simulink library "gbt_library"  (Simulink 7.4)
settings: Solver=ode45  StartTime=0.0  StopTime=10.0  RelTol=1e-3
libraries: xbsIndex_r4 x1525, casper_library_flow_control x20, casper_library_misc x15, xps_library x1
(part 1 of 14)
settings Model: Creator=mwagner  LastModifiedBy=chenhong

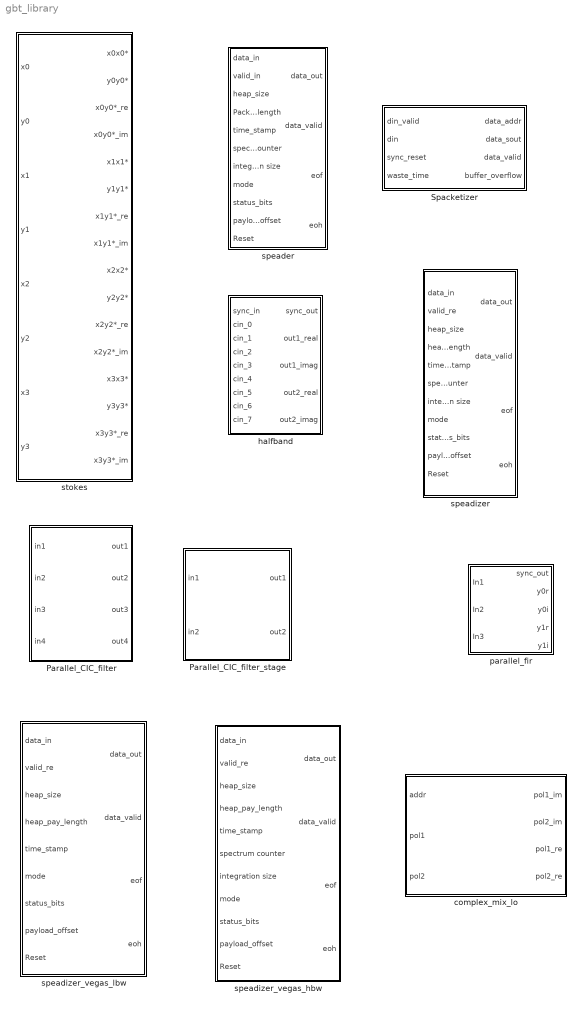
== system gbt_library ==
  Parallel_CIC_filter : Subsystem  mask(Parallel_CIC_filter){n_stages=3, dec_rate=6, n_inputs=4, polyphase=off, add_latency=1, n_bits=8, bin_pt=7, dec2_halfout=off, half2first=off, recursives=[0 1 1 1], reduced_crtc_path=off}
      mask prompts: n_stages "CIC filter Order"; dec_rate "Decimation rate"; n_inputs "Number of inputs"; polyphase "polyphase structure?(Effective only when n_inputs = 1 or n_inputs = dec_rate)"; add_latency "Add latency"; n_bits "Input bit width"; bin_pt "Binary point"; dec2_halfout "When dec_rate =2, half the number of outputs?"; half2first "Order of stages: Smaller prime factors first?"; recursives "Recursive structure for each prime-factor stage"; reduced_crtc_path "In recursive stages, invoke reduced critical path structure?"
      mask help:
      | A non-recursive CIC filter with parallel inputs.
      | Decimation rate is factored into prime numbers. Each implemented using a single stage.
      |
      | Expecting a 1-dimensional boolean vector for
      | choosing the recursive/nonrecursive structure of each prime-factor stage.
      | ([0 1 1 0] means [non-recursive recursive recursive non-recursive] stages.)
      |
      | For each stages:
      | Only supports decimation rate that is a prime number.
      | If dec_rate = 2, then we can choose n_outputs = 0.5*n_inputs(less resource)
      |     or n_outputs = n_inputs.
      | In other cases, n_outputs = n_inputs.
      | Polyphase structure available for stages of n_inputs is 1 or 2.
      mask init:
      | config.source = str2func('parallel_cic_filter_init_xblock');
      | config.toplevel = gcb;
      | config.depend = get_dependlist('parallel_cic_filter'); 
      | set_param(gcb,'LinkStatus','inactive');
      | xBlock(config, {config.toplevel,...
      |                 'n_stages',n_stages, ...
      |                 'dec_rate', dec_rate, ...
      |                 'n_inputs', n_inputs,...
      |                 'polyphase', polyphase,...
      |                 'add_latency',add_latency,...
      |                 'dec2_halfout', dec2_halfout, ...
      |                 'half2first', half2first,...
      |                 'n_bits', n_bits, ...
      |                 'bin_pt', bin_pt,...
      |                 'reduced_crtc_path', reduced_crtc_path, ...
      |                 'recursives', recursives} ...
      |                 );
      | disp('new block added');
      settings: AttributesFormatString=|
      | dec_rate = 6
      | Order = 3
  Parallel_CIC_filter_stage : Subsystem  mask(Parallel_CIC_filter_stage){n_stages=3, dec_rate=3, n_inputs=2, polyphase=off, add_latency=1, n_bits=8, bin_pt=7, dec2_halfout=on, recursive=on, reduced_crtc_path=on}
      mask prompts: n_stages "CIC filter Order"; dec_rate "Decimation rate"; n_inputs "Number of Inputs"; polyphase "polyphase structure?(Effective only when n_inputs = 1 or n_inputs = dec_rate)"; add_latency "Add latency"; n_bits "Input bit width"; bin_pt "Binary point"; dec2_halfout "When dec_rate =2, half the number of outputs?"; recursive "Recursive Structure?"; reduced_crtc_path "In recursive stages, invoke reduced critical path structure?"
      mask help:
      | A single stage of CIC filter with parallel inputs.
      | Only supports decimation rate that is a prime number.
      | If dec_rate = 2, then n_outputs = 0.5*n_inputs.
      | In other cases, n_outputs = n_inputs.
      | Polyphase structure available when n_inputs is 1 or 2.
      mask init:
      | config.source=str2func('parallel_polynomial_dec_stage_init_xblock');
      | config.toplevel=gcb;
      | config.depend = get_dependlist('parallel_polynomial_dec_stage');
      | set_param(gcb,'LinkStatus','inactive');
      | xBlock(config, {config.toplevel, ...
      |                 'n_stages', n_stages, ...
      |                 'dec_rate', dec_rate, ...
      |                 'n_inputs', n_inputs, ...
      |                 'polyphase', polyphase, ...
      |                 'add_latency', add_latency, ...
      |                 'n_bits', n_bits, ...
      |                 'bin_pt', bin_pt, ...
      |                 'dec2_halfout', dec2_halfout, ...
      |                 'recursive', recursive, ...
      |                 'reduced_crtc_path', reduced_crtc_path});
      settings: AttributesFormatString=|
      | recursive
      |  8_in
      |  reducded critical path: off
      mask CallbackString:
      | |n=get_param(gcb,'dec_rate');
      | if ~isempty(n)
      |     n = eval(n);
      |     if ~isprime(n)
      |         errordlg('Only supports decimation rate that is a prime number');
      |         set_param(gcb,'dec_rate','');
      |     end
      | end||||||||
  Spacketizer : Subsystem  AncestorBlock=gbt_library/packetizer  mask(packetizer){pin_width=256, sout_width=64, fifo_depth=128, total_words=32}
      mask prompts: pin_width "Parallel Input Width"; sout_width "Serial Output Width"; fifo_depth "FIFO depth"; total_words "Total number of data points"
      mask help:
      | This block is intended to serialize data that is 'bursty', that is,
      | the average data rate is small but per cycle the data is highly
      | parallel and can contain many points simultaneously.  This situation
      | is common with the streaming CASPER FFTs and related blocks.
      |
      | The serialization buffers the data when valid and independently
      | serializes the data when the buffer is non-empty.  For convenience, the
      | data is counted as it is serialized and signals exist to indicate
      | that the serial output is valid or that a buffer overflow has occured.  The
      | block will not stop in the case of an overflow, and the overflow
      | signal is not held high after it occurs.
      |
      | For example usage, see 'roach_spec_2adc_borph' in 'SVNROOT/trunk/projects/roach_spec/'
      | or the test case in 'SVNROOT/trunk/mlib_devel_10_1/Tests/packetizer_test.mdl'
      |
      | For extended documentation, please see the CASPER wiki
      mask init:
      | packetizer_init(gcb, 'pin_width', pin_width, 'sout_width', sout_width, 'total_words', total_words, 'fifo_depth', fifo_depth)
      | % packetizer_init(gcb, ...
      | %     'pin_width', pin_width, ...
      | %     'sout_width', sout_width, ...
      | %   %  'fifo_depth', fifo_depth, ...
      | %     'total_words', total_words);
      settings: AttributesFormatString=|
      | Parallel Input Width: 256
      | Serial Output Width: 64
      mask StyleString: edit,edit,popup(16|32|64|128|256|512|1K|2K|4K|8K|16K|32K|64K),edit
  complex_mix_lo : Subsystem  AncestorBlock=gbt_library/complex_mix_lo
  halfband : Subsystem  mask(halfband filter){ExplicitCoefficient=off, filter_coeffs=0, n_taps=4, window=hamming}
      mask prompts: ExplicitCoefficient "Explicitly define coefficients?"; filter_coeffs "Filter Coefficients"; n_taps "Number of Taps (FIR order)"; window "Window Type"
      mask help: A halfband filter for 8 complex inputs
      mask init:
      | config.source = str2func('half_band_init_xblock');
      | config.depend = get_dependlist('half_band');
      | config.debug = 0;
      | config.toplevel = gcb;
      | disp('hey');
      | ExplicitCoefficient
      | filter_coeffs
      | n_taps
      | window
      | xBlock(config, {config.toplevel, ...
      |                  'ExplicitCoefficient', ExplicitCoefficient, ...
      |                  'filter_coeffs', filter_coeffs, ...
      |                  'n_taps', n_taps, ...
      |                  'window', window, ...
      |     });
      mask Help: eval('xlWeb(''http://casper.berkeley.edu/wiki/halfband'')')
      mask StyleString: checkbox,edit,edit,popup(hamming|chebwin|gausswin|kaiserwin)
      mask CallbackString:
      | e_c = get_param(gcb, 'ExplicitCoefficient');
      | if strcmp(e_c, 'off')
      |     n_e_c = 'on';
      | else
      |     n_e_c = 'off';
      | end
      | set_param_state(gcb, 'filter_coeffs', e_c);
      | set_param_state(gcb, 'n_taps', n_e_c);
      | set_param_state(gcb, 'window', n_e_c);|||
  parallel_fir : Subsystem  mask(Parallel FIR Filter){filter_coeffs=[1 2 3 4 5 6 7 8]}
      mask prompts: filter_coeffs "Filter coefficients"
      mask help: Xblock
      mask init:
      | config.source=str2func('parallel_fir_init_xblock');
      | config.toplevel=gcb;
      | config.depend = get_dependlist('parallel_fir');
      | set_param(gcb,'LinkStatus','inactive');
      | xBlock(config, ...
      |         {config.toplevel, filter_coeffs})
      mask CallbackString:
      | filter_coeffs = get_param(gcb,'filter_coeffs');
      | if ~isempty(filter_coeffs)
      |     filter_coeffs = eval(filter_coeffs);
      |     if parallel_fir_coefficient_check(filter_coeffs)
      |         set_param(gcb,'filter_coeffs','');
      |     end
      | end
  speader : Subsystem  AncestorBlock=gbt_library/spead_packet  mask{spead_msw=64, spead_lsw=40, num_items=6, num_payloads=2}
      mask prompts: num_items "Number of items (+5)"; num_payloads "number of payloads"
      mask help:
      | The size of the heap and payload are in Bytes.
      | If there is one packet per heap then payload_offset is 0.
      | All the input must be not longer than 40 bits.
  speadizer : Subsystem  AncestorBlock=gbt_library/spead_packet  mask{spead_msw=64, spead_lsw=40, num_items=6, num_payloads=2}
      mask prompts: num_items "Number of items (+5)"; num_payloads "number of payloads"
      mask help:
      | The size of the heap and payload are in Bytes.
      | If there is one packet per heap then payload_offset is 0.
      | All the input must be not longer than 40 bits.
  speadizer_vegas_hbw : Subsystem  AncestorBlock=gbt_library/speadizer  mask(speadizer_vegas){spead_msw=64, spead_lsw=40, num_items=6, num_payloads=2, pktzr_waste_time=7, data_input_width=512}
      mask prompts: spead_msw "Num bits for SPEAD Item ID"; spead_lsw "Num bits for SPEAD Item value"; num_items "Number of items (+5)"; num_payloads "Number of packets per heap"; pktzr_waste_time "Packetizer waste time"; data_input_width "Data input width"
      mask help:
      | The size of the heap and payload are in Bytes.
      | If there is one packet per heap then payload_offset is 0.
      | All the input must be not longer than 40 bits.
      mask init:
      | speadizer_vegas_init(gcb, 'spead_msw', spead_msw, 'spead_lsw', spead_lsw, 'num_items', num_items, 'num_payloads', num_payloads, 'pktzr_waste_time', pktzr_waste_time, 'data_input_width', data_input_width)
  speadizer_vegas_lbw : Subsystem  mask(speadizer_vegas){spead_msw=24, spead_lsw=40, num_items=4, num_payloads=1, pktzr_waste_time=0, data_input_width=256}
      mask prompts: spead_msw "Num bits for SPEAD Item ID"; spead_lsw "Num bits for SPEAD Item value"; num_items "Number of items (+5)"; num_payloads "Number of packets per heap"; pktzr_waste_time "Packetizer waste time"; data_input_width "Data input width"
      mask help:
      | The size of the heap and payload are in Bytes.
      | If there is one packet per heap then payload_offset is 0.
      | All the input must be not longer than 40 bits.
      mask init: same as gbt_library/speadizer_vegas_hbw
  stokes : Subsystem  mask{n_samples=4}
      mask prompts: n_samples "Number of Simultaneous Inputs"
      mask init:
      | % To make the xBlock smart so it won''t re-generate the
      | % subsystem if neither the arguments nor the scripts are
      | % changes, use as the following:
      | cfg.source = str2func('stokes_init');
      | cfg.toplevel = gcb;
      | cfg.depend = {'stokes_init'};
      | args = {n_samples};
      | xBlock(cfg, args);
      mask TabNameString: Basic

== system gbt_library/Parallel_CIC_filter ==
  in1 : Inport
  in2 : Inport  Port=2
  in3 : Inport  Port=3
  in4 : Inport  Port=4
  Stage1_dec3 : Subsystem
      settings: AttributesFormatString=|
      | nonrecursive
      | 8_in
      | polyphase:off
  Stage2_dec2 : Subsystem
      settings: AttributesFormatString=|
      | recursive
      | 13_in
      | reduced critical path structureoff
  out1 : Outport
  out2 : Outport  Port=2
  out3 : Outport  Port=3
  out4 : Outport  Port=4
  wires:
  Stage2_dec2/4(out4) -> out4/1
  Stage2_dec2/3(out3) -> out3/1
  Stage2_dec2/2(out2) -> out2/1
  Stage2_dec2/1(out1) -> out1/1
  Stage1_dec3/4(out4) -> Stage2_dec2/4(in4)  "sig2_4"
  Stage1_dec3/3(out3) -> Stage2_dec2/3(in3)  "sig2_3"
  Stage1_dec3/2(out2) -> Stage2_dec2/2(in2)  "sig2_2"
  Stage1_dec3/1(out1) -> Stage2_dec2/1(in1)  "sig2_1"
  in4/1 -> Stage1_dec3/4(in4)
  in3/1 -> Stage1_dec3/3(in3)
  in2/1 -> Stage1_dec3/2(in2)
  in1/1 -> Stage1_dec3/1(in1)

== system gbt_library/Parallel_CIC_filter_stage ==
  in1 : Inport
  in2 : Inport  Port=2
  comb_1 : Subsystem
      settings: AttributesFormatString=|
      | Differentiation length = 1
      | Bitwidth = 13 bin_pt=7
  comb_2 : Subsystem
      settings: AttributesFormatString=|
      | Differentiation length = 1
      | Bitwidth = 13 bin_pt=7
  comb_3 : Subsystem
      settings: AttributesFormatString=|
      | Differentiation length = 1
      | Bitwidth = 13 bin_pt=7
  downsample_3 : Subsystem
      settings: AttributesFormatString=Decimation Rate = 3
  int_1 : Subsystem
      settings: AttributesFormatString=|
      | Add Latency = 1
      | Bitwidth = 13 bin_pt = 7
  int_2 : Subsystem
      settings: AttributesFormatString=|
      | Add Latency = 1
      | Bitwidth = 13 bin_pt = 7
  int_3 : Subsystem
      settings: AttributesFormatString=|
      | Add Latency = 1
      | Bitwidth = 13 bin_pt = 7
  out1 : Outport
  out2 : Outport  Port=2
  wires:
  in1/1 -> downsample_3/1(sync_in), int_1/3(sync), int_1/1(in1)
  int_1/1(out1) -> int_2/3(sync), int_2/1(in1)  "int_ins1_1"
  int_2/1(out1) -> int_3/3(sync), int_3/1(in1)  "int_ins2_1"
  comb_3/3(out2) -> out2/1  "comb_ins3_2"
  comb_3/2(out1) -> out1/1  "comb_ins3_1"
  comb_2/3(out2) -> comb_3/3(in2)  "comb_ins2_2"
  comb_2/2(out1) -> comb_3/2(in1)  "comb_ins2_1"
  comb_2/1(sync_out) -> comb_3/1(sync_in)  "comb_sync_in3"
  comb_1/3(out2) -> comb_2/3(in2)  "comb_ins1_2"
  comb_1/2(out1) -> comb_2/2(in1)  "comb_ins1_1"
  comb_1/1(sync_out) -> comb_2/1(sync_in)  "comb_sync_in2"
  downsample_3/3(Out2) -> comb_1/3(in2)  "ds_out2"
  downsample_3/2(Out1) -> comb_1/2(in1)  "ds_out1"
  downsample_3/1(sync_out) -> comb_1/1(sync_in)  "ds_sync_out"
  int_3/2(out2) -> downsample_3/3(In2)  "int_ins3_2"
  int_3/1(out1) -> downsample_3/2(In1)  "int_ins3_1"
  int_2/2(out2) -> int_3/2(in2)  "int_ins2_2"
  int_1/2(out2) -> int_2/2(in2)  "int_ins1_2"
  in2/1 -> int_1/2(in2)

== system gbt_library/Spacketizer ==
  din_valid : Inport
  din : Inport  Port=2
  sync_reset : Inport  Port=3
  waste_time : Inport  Port=4
  Counter : xbsIndex_r4/Counter  cnt_type=Free Running  cnt_to=Inf  operation=Up  start_count=0  cnt_by_val=1  arith_type=Unsigned  n_bits=11  bin_pt=0  load_pin=off  rst=on  en=on  explicit_period=on  period=1  dbl_ovrd=off  use_behavioral_HDL=off  implementation=Fabric  use_rpm=off  block_type=counter
  Inverter : xbsIndex_r4/Inverter  en=off  latency=0  dbl_ovrd=off  block_type=inv
  Logical : xbsIndex_r4/Logical  logical_function=AND  inputs=2  en=off  latency=0  precision=Full  arith_type=Unsigned  n_bits=16  bin_pt=0  align_bp=on  dbl_ovrd=off  block_type=logical
  Logical1 : xbsIndex_r4/Logical  logical_function=AND  inputs=2  en=off  latency=0  precision=Full  arith_type=Unsigned  n_bits=16  bin_pt=0  align_bp=on  dbl_ovrd=off  block_type=logical
  data_buffer : xbsIndex_r4/FIFO  depth=128  percent_nbits=1  rst=off  en=off  use_dcount=off  use_almost_empty=off  almost_empty_thresh=2  use_almost_full=off  almost_full_thresh=14  dbl_ovrd=off  mem_type=Block RAM  explicit_period=off  block_type=fifo
      settings: block_version=10.1.3
  data_counter : xbsIndex_r4/Counter  cnt_type=Free Running  cnt_to=Inf  operation=Up  start_count=0  cnt_by_val=1  arith_type=Unsigned  n_bits=6  bin_pt=0  load_pin=off  rst=on  en=on  explicit_period=on  period=1  dbl_ovrd=off  use_behavioral_HDL=off  implementation=Fabric  use_rpm=off  block_type=counter
  packetizer_fsm : xbsIndex_r4/MCode  mfname=packetizer_fsm  explicit_period=off  period=1  inputsTable={'boundInpExpr'=>['','','3','','31','','',''],'inputs'=>['fifo_empty','shift_count','data_per_word','data_count','n_words','sync_reset','waste_count','waste_time']}  outputsTable={'outputs'=>['fifo_re','bram_addr_en','bram_we','serializer_shift','serializer_ld','shift_count_en','shift_count_rst','bram_addr_rst','data_count_en','data_count_rst','done','waste_count_en','waste_count_rst'],'suppressOut'=>['off','off','off','off','off','off','off','off','off','off','off','off','off']}  dbl_ovrd=off  enable_stdout=off  enable_debug=off  suppress_output=on  defparams={'data_per_word',3,'n_words',31}  hide_port_list={}  block_type=mcode
      settings: block_version=11.4
  parallel_to_serial_converter : Subsystem  AncestorBlock=casper_library/Flow_Control/parallel_to_serial_converter  mask(parallel_to_serial_converter){pin_width=256, sout_width=64}
      mask prompts: pin_width "Parallel Input Width"; sout_width "Serial Output Width"
      mask help:
      | This block takes as input a parallel bus of specified width.
      | When the load signal 'ld' is asserted, this data is broken into
      | pieces of width specified by the serial output width and
      | stored into different registers chained to form a shift register.
      | If the 'shift' input is subsequently asserted, the shift register
      | returns as output a new piece of data of width sout_width.  This data
      | is the next least significant piece of the original bus.  The converter
      | serializes SMALL ENDIAN.
      |
      | Note that the load operation automatically loads the least significant
      | bits into the register closest to the output, so the first 'shift'
      | assertion changes the data output from bits [sout_width-1:0] to
      | bits [2*sout_width-1:sout_width].
      mask init:
      | parallel_to_serial_converter_init(gcb, ...
      |     'pin_width', pin_width, ...
      |     'sout_width', sout_width);
  shift_counter : xbsIndex_r4/Counter  cnt_type=Free Running  cnt_to=Inf  operation=Up  start_count=0  cnt_by_val=1  arith_type=Unsigned  n_bits=3  bin_pt=0  load_pin=off  rst=on  en=on  explicit_period=on  period=1  dbl_ovrd=off  use_behavioral_HDL=off  implementation=Fabric  use_rpm=off  block_type=counter
  waste_counter : xbsIndex_r4/Counter  cnt_type=Free Running  cnt_to=Inf  operation=Up  start_count=0  cnt_by_val=1  arith_type=Unsigned  n_bits=5  bin_pt=0  load_pin=off  rst=on  en=on  explicit_period=on  period=1  dbl_ovrd=off  use_behavioral_HDL=off  implementation=Fabric  use_rpm=off  block_type=counter
  data_addr : Outport
  data_sout : Outport  Port=2
  data_valid : Outport  Port=3
  buffer_overflow : Outport  Port=4
  wires:
  waste_time/1 -> packetizer_fsm/6
  packetizer_fsm/13 -> waste_counter/1
  packetizer_fsm/12 -> waste_counter/2
  waste_counter/1 -> packetizer_fsm/5
  sync_reset/1 -> packetizer_fsm/4
  packetizer_fsm/10 -> data_counter/1
  data_counter/1 -> packetizer_fsm/3
  packetizer_fsm/9 -> data_counter/2
  packetizer_fsm/8 -> Counter/1
  packetizer_fsm/2 -> Counter/2
  Counter/1 -> data_addr/1
  data_buffer/2 -> packetizer_fsm/1
  packetizer_fsm/7 -> shift_counter/1
  shift_counter/1 -> packetizer_fsm/2
  packetizer_fsm/6 -> shift_counter/2
  parallel_to_serial_converter/1(sout) -> data_sout/1
  din/1 -> data_buffer/1
  packetizer_fsm/3 -> data_valid/1
  packetizer_fsm/5 -> parallel_to_serial_converter/2(ld)
  packetizer_fsm/4 -> parallel_to_serial_converter/3(shift)
  packetizer_fsm/1 -> data_buffer/3
  data_buffer/1 -> parallel_to_serial_converter/1(pin)
  Logical/1 -> data_buffer/2
  din_valid/1 -> Logical/1, Logical1/1
  Inverter/1 -> Logical/2
  data_buffer/4 -> Inverter/1, Logical1/2
  Logical1/1 -> buffer_overflow/1

== system gbt_library/complex_mix_lo ==
  addr : Inport
  pol1 : Inport  Port=2
  pol2 : Inport  Port=3
  Constant10 : xbsIndex_r4/Constant  arith_type=Unsigned  const=0  n_bits=18  bin_pt=0  explicit_period=on  period=1  equ=P=C  opselect=C  inp2=PCIN>>17  opr=+  inp1=P  carry=CIN  dbl_ovrd=off  block_type=constant
  Constant9 : xbsIndex_r4/Constant  arith_type=Unsigned  const=0  n_bits=18  bin_pt=0  explicit_period=on  period=1  equ=P=C  opselect=C  inp2=PCIN>>17  opr=+  inp1=P  carry=CIN  dbl_ovrd=off  block_type=constant
  Mult{1..3,16} (4 alike) : xbsIndex_r4/Mult  precision=Full  arith_type="Signed  (2's comp)"  n_bits=16  bin_pt=14  quantization=Truncate  overflow=Wrap  en=off  latency=3  dbl_ovrd=off  use_behavioral_HDL=off  opt=Speed  use_embedded=on  optimum_pipeline=off  pipeline=on  use_rpm=on  placement_style=Triangular  block_type=mult
      settings: block_version=11.4
  Reinterpret12 : xbsIndex_r4/Reinterpret  force_arith_type=on  arith_type="Signed  (2's comp)"  force_bin_pt=on  bin_pt=15  block_type=reinterpret
      settings: infoedit="Changes signal type without altering the binary representation.   You can changed the signal between signed and unsigned, and relocate the binary point.<br><br>Hardware notes: In hardware this block costs nothing.<br><br>Example:  Suppose the input is 6 bits wide, signed, with 2 fractional bits, and the output is forced to unsigned with 0 fractional bits.  Then an input of -2.0 (1110.00 in binary 2's complement) becomes an output of 56 (111000 in binary)."
  Reinterpret9 : xbsIndex_r4/Reinterpret  force_arith_type=on  arith_type="Signed  (2's comp)"  force_bin_pt=on  bin_pt=15  block_type=reinterpret
      settings: infoedit="Changes signal type without altering the binary representation.   You can changed the signal between signed and unsigned, and relocate the binary point.<br><br>Hardware notes: In hardware this block costs nothing.<br><br>Example:  Suppose the input is 6 bits wide, signed, with 2 fractional bits, and the output is forced to unsigned with 0 fractional bits.  Then an input of -2.0 (1110.00 in binary 2's complement) becomes an output of 56 (111000 in binary)."
  cos_slice4 : xbsIndex_r4/Slice  nbits=16  boolean_output=off  mode=Lower Bit Location + Width  bit1=0  base1=MSB of Input  bit0=0  base0=LSB of Input  dbl_ovrd=off  block_type=slice
  delay{32..39,80..83} (12 alike) : xbsIndex_r4/Delay  en=off  latency=1  dbl_ovrd=off  reg_retiming=on  block_type=delay
      settings: block_version=11.4
  lo_ram : xps_library/Shared BRAM  Tag=xps:bram  SystemSampleTime=-1  arith_type="Signed  (2's comp)"  addr_width=11  data_width=32  data_bin_pt=0  init_vals=[1:2^11]  sample_rate=1
  sin_slice4 : xbsIndex_r4/Slice  nbits=16  boolean_output=off  mode=Upper Bit Location + Width  bit1=0  base1=MSB of Input  bit0=0  base0=LSB of Input  dbl_ovrd=off  block_type=slice
  pol1_im : Outport
  pol2_im : Outport  Port=2
  pol1_re : Outport  Port=3
  pol2_re : Outport  Port=4
  wires:
  addr/1 -> lo_ram/1
  pol1/1 -> delay36/1, delay32/1
  delay83/1 -> pol2_re/1
  delay82/1 -> pol1_re/1
  delay81/1 -> pol2_im/1
  pol2/1 -> delay38/1, delay34/1
  delay80/1 -> pol1_im/1
  delay39/1 -> Mult3/2
  delay38/1 -> Mult3/1
  delay37/1 -> Mult2/2
  delay36/1 -> Mult2/1
  delay35/1 -> Mult1/2
  delay34/1 -> Mult1/1
  delay33/1 -> Mult16/2
  delay32/1 -> Mult16/1
  Mult3/1 -> delay83/1
  cos_slice4/1 -> Reinterpret9/1
  Reinterpret9/1 -> delay39/1, delay37/1
  Mult2/1 -> delay82/1
  Mult1/1 -> delay81/1
  lo_ram/1 -> sin_slice4/1, cos_slice4/1
  sin_slice4/1 -> Reinterpret12/1
  Reinterpret12/1 -> delay35/1, delay33/1
  Mult16/1 -> delay80/1
  Constant10/1 -> lo_ram/2
  Constant9/1 -> lo_ram/3

== system gbt_library/halfband ==
  sync_in : Inport
  cin_0 : Inport  Port=2
  cin_1 : Inport  Port=3
  cin_2 : Inport  Port=4
  cin_3 : Inport  Port=5
  cin_4 : Inport  Port=6
  cin_5 : Inport  Port=7
  cin_6 : Inport  Port=8
  cin_7 : Inport  Port=9
  adder_tree : Subsystem
      settings: AttributesFormatString=latency 2
  adder_tree1 : Subsystem
      settings: AttributesFormatString=latency 2
  adder_tree3 : Subsystem
      settings: AttributesFormatString=latency 2
  adder_tree4 : Subsystem
      settings: AttributesFormatString=latency 2
  parallel_fir : Subsystem
      settings: AttributesFormatString=8_7 r/i
  parallel_fir1 : Subsystem
      settings: AttributesFormatString=8_7 r/i
  parallel_fir2 : Subsystem
      settings: AttributesFormatString=8_7 r/i
  parallel_fir3 : Subsystem
      settings: AttributesFormatString=8_7 r/i
  sync_out : Outport
  out1_real : Outport  Port=2
  out1_imag : Outport  Port=3
  out2_real : Outport  Port=4
  out2_imag : Outport  Port=5
  wires:
  sync_in/1 -> parallel_fir3/1(sync_in), parallel_fir2/1(sync_in), parallel_fir1/1(sync_in), parallel_fir/1(sync_in)
  parallel_fir/1(sync_out) -> adder_tree4/1(sync), adder_tree3/1(sync), adder_tree1/1(sync), adder_tree/1(sync)  "dec_fir_sync_out"
  parallel_fir3/5(y1i) -> adder_tree4/5(din4)  "imag_v7_out"
  parallel_fir3/4(y1r) -> adder_tree3/5(din4)  "real_v7_out"
  parallel_fir3/3(y0i) -> adder_tree1/5(din4)  "imag_v3_out"
  parallel_fir3/2(y0r) -> adder_tree/5(din4)  "real_v3_out"
  cin_7/1 -> parallel_fir3/3(in2)
  cin_3/1 -> parallel_fir3/2(in1)
  parallel_fir2/5(y1i) -> adder_tree4/4(din3)  "imag_v6_out"
  parallel_fir2/4(y1r) -> adder_tree3/4(din3)  "real_v6_out"
  parallel_fir2/3(y0i) -> adder_tree1/4(din3)  "imag_v2_out"
  parallel_fir2/2(y0r) -> adder_tree/4(din3)  "real_v2_out"
  cin_6/1 -> parallel_fir2/3(in2)
  cin_2/1 -> parallel_fir2/2(in1)
  parallel_fir1/5(y1i) -> adder_tree4/3(din2)  "imag_v5_out"
  parallel_fir1/4(y1r) -> adder_tree3/3(din2)  "real_v5_out"
  parallel_fir1/3(y0i) -> adder_tree1/3(din2)  "imag_v1_out"
  parallel_fir1/2(y0r) -> adder_tree/3(din2)  "real_v1_out"
  cin_5/1 -> parallel_fir1/3(in2)
  cin_1/1 -> parallel_fir1/2(in1)
  parallel_fir/5(y1i) -> adder_tree4/2(din1)  "imag_v4_out"
  parallel_fir/4(y1r) -> adder_tree3/2(din1)  "real_v4_out"
  parallel_fir/3(y0i) -> adder_tree1/2(din1)  "imag_v0_out"
  parallel_fir/2(y0r) -> adder_tree/2(din1)  "real_v0_out"
  cin_4/1 -> parallel_fir/3(in2)
  cin_0/1 -> parallel_fir/2(in1)
  adder_tree4/2(dout) -> out2_imag/1
  adder_tree3/2(dout) -> out2_real/1
  adder_tree1/2(dout) -> out1_imag/1
  adder_tree/2(dout) -> out1_real/1
  adder_tree/1(sync_out) -> sync_out/1

== system gbt_library/parallel_fir ==
  In1 : Inport
  In2 : Inport  Port=2
  In3 : Inport  Port=3
  AddSub{1,3,5..6} (4 alike) : xbsIndex_r4/AddSub  mode=Subtraction  use_carryin=off  use_carryout=off  en=off  latency=0  precision=Full  arith_type=Unsigned  n_bits=16  bin_pt=14  quantization=Truncate  overflow=Wrap  dbl_ovrd=off  use_behavioral_HDL=off  hw_selection=Fabric  pipelined=off  block_type=addsub
  AddSub2 : xbsIndex_r4/AddSub  mode=Addition  use_carryin=off  use_carryout=off  en=off  latency=0  precision=Full  arith_type=Unsigned  n_bits=16  bin_pt=14  quantization=Truncate  overflow=Wrap  dbl_ovrd=off  use_behavioral_HDL=off  hw_selection=Fabric  pipelined=off  block_type=addsub
  AddSub4 : xbsIndex_r4/AddSub  mode=Addition  use_carryin=off  use_carryout=off  en=off  latency=0  precision=Full  arith_type=Unsigned  n_bits=16  bin_pt=14  quantization=Truncate  overflow=Wrap  dbl_ovrd=off  use_behavioral_HDL=off  hw_selection=Fabric  pipelined=off  block_type=addsub
  Delay : xbsIndex_r4/Delay  en=off  latency=1  dbl_ovrd=off  reg_retiming=off  block_type=delay
      settings: block_version=11.4
  Delay1 : xbsIndex_r4/Delay  en=off  latency=1  dbl_ovrd=off  reg_retiming=off  block_type=delay
      settings: block_version=11.4
  c_to_ri : Subsystem
      settings: AttributesFormatString=8_7 r/i
  c_to_ri1 : Subsystem
      settings: AttributesFormatString=8_7 r/i
  c_to_ri2 : Subsystem
      settings: AttributesFormatString=8_7 r/i
  f0 : Subsystem
      settings: AttributesFormatString=|
      | 4 taps
      | 4_3 r/i
  f0pf1 : Subsystem
      settings: AttributesFormatString=|
      | 4 taps
      | 4_3 r/i
  f1 : Subsystem
      settings: AttributesFormatString=|
      | 4 taps
      | 4_3 r/i
  sync_out : Outport
  y0r : Outport  Port=2
  y0i : Outport  Port=3
  y1r : Outport  Port=4
  y1i : Outport  Port=5
  wires:
  c_to_ri/1(re) -> AddSub5/1, AddSub2/1
  c_to_ri/2(im) -> AddSub6/1, AddSub4/1
  c_to_ri2/1(re) -> Delay/1, AddSub1/2
  c_to_ri2/2(im) -> Delay1/1, AddSub3/2
  In1/1 -> f1/1(sync_in), f0pf1/1(sync_in), f0/1(sync_in)
  In2/1 -> f1/2(real1), f0pf1/2(real1), f0/2(real1)
  In3/1 -> f1/3(imag1), f0pf1/3(imag1), f0/3(imag1)
  f1/2(dout) -> c_to_ri2/1(c)
  f0pf1/2(dout) -> c_to_ri1/1(c)
  f0/2(dout) -> c_to_ri/1(c)
  f0/1(sync_out) -> sync_out/1
  c_to_ri1/2(im) -> AddSub3/1
  c_to_ri1/1(re) -> AddSub1/1
  Delay1/1 -> AddSub4/2
  Delay/1 -> AddSub2/2
  AddSub6/1 -> y1i/1
  AddSub3/1 -> AddSub6/2
  AddSub5/1 -> y1r/1
  AddSub1/1 -> AddSub5/2
  AddSub4/1 -> y0i/1
  AddSub2/1 -> y0r/1

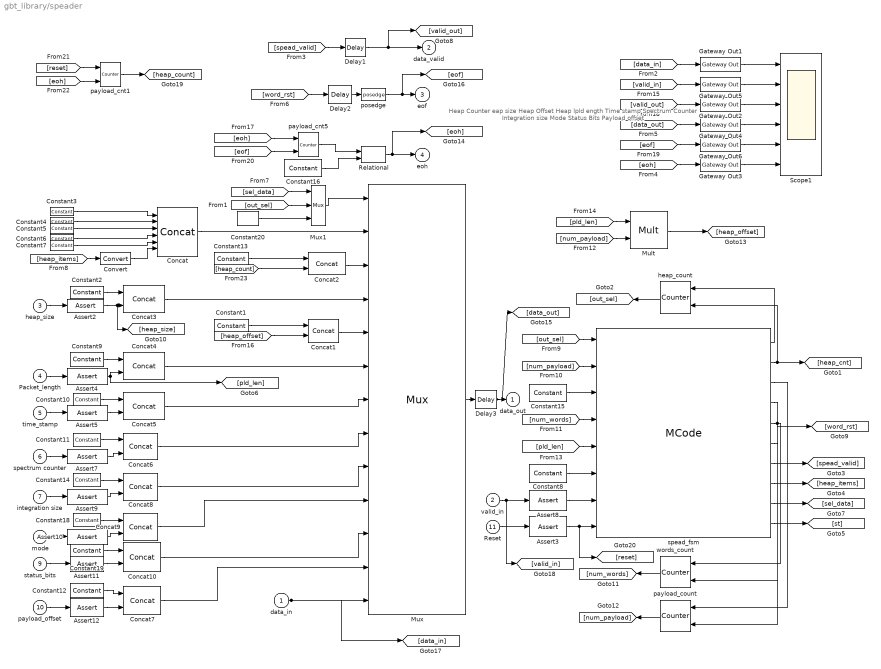
== system gbt_library/speader ==
  note: Heap Counter
      | eap size
      | Heap Offset
      | Heap lpld ength
      | Time stamp
      | Spectrum Counter
      | Integration size
      | Mode
      | Status Bits
      | Payload offset
  data_in : Inport
  valid_in : Inport  Port=2
  heap_size : Inport  Port=3
  Packet_length : Inport  Port=4
  time_stamp : Inport  Port=5
  spectrum counter : Inport  Port=6
  integration size : Inport  Port=7
  mode : Inport  Port=8
  status_bits : Inport  Port=9
  payload_offset : Inport  Port=10
  Reset : Inport  Port=11
  Assert{2,4..5,7,9..12} (8 alike) : xbsIndex_r4/Assert  assert_type=on  type_source=Explicitly  arith_type=Unsigned  n_bits=spead_lsw  bin_pt=0  assert_rate=off  rate_source=Explicitly  period=1  output_port=on  block_type=assert
      settings: block_version=11.4
  Assert3 : xbsIndex_r4/Assert  assert_type=on  type_source=Explicitly  arith_type=Boolean  n_bits=spead_lsw  bin_pt=0  assert_rate=on  rate_source=Explicitly  period=1  output_port=on  block_type=assert
      settings: block_version=11.4
  Assert8 : xbsIndex_r4/Assert  assert_type=on  type_source=Explicitly  arith_type=Boolean  n_bits=spead_lsw  bin_pt=0  assert_rate=on  rate_source=Explicitly  period=1  output_port=on  block_type=assert
      settings: block_version=11.4
  Concat : xbsIndex_r4/Concat  num_inputs=6  dbl_ovrd=off  block_type=concat
  Concat{1..10} (10 alike) : xbsIndex_r4/Concat  num_inputs=2  dbl_ovrd=off  block_type=concat
  Constant1 : xbsIndex_r4/Constant  arith_type=Unsigned  const=8388608+3  n_bits=spead_msw-spead_lsw  bin_pt=0  explicit_period=on  period=1  equ=P=C  opselect=C  inp2=PCIN>>17  opr=+  inp1=P  carry=CIN  dbl_ovrd=off  block_type=constant
      settings: block_version=11.4
  Constant10 : xbsIndex_r4/Constant  arith_type=Unsigned  const=8388608+32  n_bits=spead_msw-spead_lsw  bin_pt=0  explicit_period=on  period=1  equ=P=C  opselect=C  inp2=PCIN>>17  opr=+  inp1=P  carry=CIN  dbl_ovrd=off  block_type=constant
      settings: block_version=11.4
  Constant11 : xbsIndex_r4/Constant  arith_type=Unsigned  const=8388608+33  n_bits=spead_msw-spead_lsw  bin_pt=0  explicit_period=on  period=1  equ=P=C  opselect=C  inp2=PCIN>>17  opr=+  inp1=P  carry=CIN  dbl_ovrd=off  block_type=constant
      settings: block_version=11.4
  Constant12 : xbsIndex_r4/Constant  arith_type=Unsigned  const=37  n_bits=spead_msw-spead_lsw  bin_pt=0  explicit_period=on  period=1  equ=P=C  opselect=C  inp2=PCIN>>17  opr=+  inp1=P  carry=CIN  dbl_ovrd=off  block_type=constant
      settings: block_version=11.4
  Constant13 : xbsIndex_r4/Constant  arith_type=Unsigned  const=8388608+1  n_bits=spead_msw-spead_lsw  bin_pt=0  explicit_period=on  period=1  equ=P=C  opselect=C  inp2=PCIN>>17  opr=+  inp1=P  carry=CIN  dbl_ovrd=off  block_type=constant
      settings: block_version=11.4
  Constant14 : xbsIndex_r4/Constant  arith_type=Unsigned  const=8388608+34  n_bits=spead_msw-spead_lsw  bin_pt=0  explicit_period=on  period=1  equ=P=C  opselect=C  inp2=PCIN>>17  opr=+  inp1=P  carry=CIN  dbl_ovrd=off  block_type=constant
      settings: block_version=11.4
  Constant15 : xbsIndex_r4/Constant  arith_type=Unsigned  const=num_items+5  n_bits=8  bin_pt=0  explicit_period=on  period=1  equ=P=C  opselect=C  inp2=PCIN>>17  opr=+  inp1=P  carry=CIN  dbl_ovrd=off  block_type=constant
      settings: block_version=11.4
  Constant16 : xbsIndex_r4/Constant  arith_type=Unsigned  const=num_payloads  n_bits=4  bin_pt=0  explicit_period=on  period=1  equ=P=C  opselect=C  inp2=PCIN>>17  opr=+  inp1=P  carry=CIN  dbl_ovrd=off  block_type=constant
      settings: block_version=11.4
  Constant18 : xbsIndex_r4/Constant  arith_type=Unsigned  const=8388608+35  n_bits=spead_msw-spead_lsw  bin_pt=0  explicit_period=on  period=1  equ=P=C  opselect=C  inp2=PCIN>>17  opr=+  inp1=P  carry=CIN  dbl_ovrd=off  block_type=constant
      settings: block_version=11.4
  Constant19 : xbsIndex_r4/Constant  arith_type=Unsigned  const=8388608+36  n_bits=spead_msw-spead_lsw  bin_pt=0  explicit_period=on  period=1  equ=P=C  opselect=C  inp2=PCIN>>17  opr=+  inp1=P  carry=CIN  dbl_ovrd=off  block_type=constant
      settings: block_version=11.4
  Constant2 : xbsIndex_r4/Constant  arith_type=Unsigned  const=8388608+2  n_bits=spead_msw-spead_lsw  bin_pt=0  explicit_period=on  period=1  equ=P=C  opselect=C  inp2=PCIN>>17  opr=+  inp1=P  carry=CIN  dbl_ovrd=off  block_type=constant
      settings: block_version=11.4
  Constant20 : xbsIndex_r4/Constant  arith_type=Unsigned  const=num_items+5  n_bits=4  bin_pt=0  explicit_period=on  period=1  equ=P=C  opselect=C  inp2=PCIN>>17  opr=+  inp1=P  carry=CIN  dbl_ovrd=off  block_type=constant
      settings: block_version=11.4
  Constant3 : xbsIndex_r4/Constant  arith_type=Unsigned  const=83  n_bits=8  bin_pt=0  explicit_period=on  period=1  equ=P=C  opselect=C  inp2=PCIN>>17  opr=+  inp1=P  carry=CIN  dbl_ovrd=off  block_type=constant
      settings: block_version=11.4
  Constant4 : xbsIndex_r4/Constant  arith_type=Unsigned  const=4  n_bits=8  bin_pt=0  explicit_period=on  period=1  equ=P=C  opselect=C  inp2=PCIN>>17  opr=+  inp1=P  carry=CIN  dbl_ovrd=off  block_type=constant
      settings: block_version=11.4
  Constant5 : xbsIndex_r4/Constant  arith_type=Unsigned  const=3  n_bits=8  bin_pt=0  explicit_period=on  period=1  equ=P=C  opselect=C  inp2=PCIN>>17  opr=+  inp1=P  carry=CIN  dbl_ovrd=off  block_type=constant
      settings: block_version=11.4
  Constant6 : xbsIndex_r4/Constant  arith_type=Unsigned  const=5  n_bits=8  bin_pt=0  explicit_period=on  period=1  equ=P=C  opselect=C  inp2=PCIN>>17  opr=+  inp1=P  carry=CIN  dbl_ovrd=off  block_type=constant
      settings: block_version=11.4
  Constant7 : xbsIndex_r4/Constant  arith_type=Unsigned  const=0  n_bits=16  bin_pt=0  explicit_period=on  period=1  equ=P=C  opselect=C  inp2=PCIN>>17  opr=+  inp1=P  carry=CIN  dbl_ovrd=off  block_type=constant
      settings: block_version=11.4
  Constant8 : xbsIndex_r4/Constant  arith_type=Unsigned  const=num_payloads  n_bits=8  bin_pt=0  explicit_period=on  period=1  equ=P=C  opselect=C  inp2=PCIN>>17  opr=+  inp1=P  carry=CIN  dbl_ovrd=off  block_type=constant
      settings: block_version=11.4
  Constant9 : xbsIndex_r4/Constant  arith_type=Unsigned  const=8388608+4  n_bits=spead_msw-spead_lsw  bin_pt=0  explicit_period=on  period=1  equ=P=C  opselect=C  inp2=PCIN>>17  opr=+  inp1=P  carry=CIN  dbl_ovrd=off  block_type=constant
      settings: block_version=11.4
  Convert : xbsIndex_r4/Convert  arith_type=Unsigned  n_bits=16  bin_pt=0  quantization=Truncate  overflow=Wrap  latency=0  dbl_ovrd=off  pipeline=off  block_type=convert
      settings: block_version=11.4
  Delay1 : xbsIndex_r4/Delay  en=off  latency=1  dbl_ovrd=off  reg_retiming=on  block_type=delay
      settings: block_version=11.4
  Delay2 : xbsIndex_r4/Delay  en=off  latency=0  dbl_ovrd=off  reg_retiming=on  block_type=delay
      settings: block_version=11.4
  Delay3 : xbsIndex_r4/Delay  en=off  latency=1  dbl_ovrd=off  reg_retiming=on  block_type=delay
      settings: block_version=11.4
  Gateway Out{1..6} (6 alike) : xbsIndex_r4/Gateway Out  hdl_port=on  timing_constraint=None  locs_specified=off  LOCs={}  block_type=gatewayout
      settings: infoedit="Gateway out block.  Converts Xilinx fixed point inputs into ouputs of type Simulink integer, double, or fixed point.<br><br>Hardware notes:  In hardware these blocks become top level output ports or are discarded, depending on how they are configured."  block_version=11.4
  Mult : xbsIndex_r4/Mult  precision=User Defined  arith_type=Unsigned  n_bits=40  bin_pt=0  quantization=Truncate  overflow=Wrap  en=off  latency=3  dbl_ovrd=off  use_behavioral_HDL=off  opt=Speed  use_embedded=on  optimum_pipeline=off  pipeline=on  use_rpm=on  placement_style=Triangular  block_type=mult
      settings: block_version=11.4
  Mux : xbsIndex_r4/Mux  inputs=12  en=off  latency=0  precision=User Defined  arith_type=Unsigned  n_bits=64  bin_pt=0  quantization=Truncate  overflow=Wrap  dbl_ovrd=off  block_type=mux
      settings: block_version=11.4
  Mux1 : xbsIndex_r4/Mux  inputs=2  en=off  latency=0  precision=Full  arith_type="Signed  (2's comp)"  n_bits=8  bin_pt=2  quantization=Truncate  overflow=Wrap  dbl_ovrd=off  block_type=mux
      settings: block_version=11.4
  Relational : xbsIndex_r4/Relational  mode=a=b  en=off  latency=0  dbl_ovrd=off  block_type=relational
  Scope1 : Scope  NumInputPorts=6
      settings: TimeRange=1000  YMin=0~0~0~0~0~0  YMax=40~1~1~1e+19~1~20  SaveName=ScopeData2  MaxDataPoints=10000
  heap_count : xbsIndex_r4/Counter  cnt_type=Free Running  cnt_to=Inf  operation=Up  start_count=0  cnt_by_val=1  arith_type=Unsigned  n_bits=4  bin_pt=0  load_pin=off  rst=on  en=on  explicit_period=on  period=1  dbl_ovrd=off  use_behavioral_HDL=off  implementation=Fabric  block_type=counter
      settings: block_version=11.4
  payload_cnt1 : xbsIndex_r4/Counter  cnt_type=Free Running  cnt_to=0  operation=Up  start_count=1024  cnt_by_val=1  arith_type=Unsigned  n_bits=40  bin_pt=0  load_pin=off  rst=on  en=on  explicit_period=on  period=1  dbl_ovrd=off  use_behavioral_HDL=off  implementation=Fabric  use_rpm=on  block_type=counter
      settings: xl_area=[0, 0, 0, 0, 0, 0, 0]
  payload_cnt5 : xbsIndex_r4/Counter  cnt_type=Free Running  cnt_to=0  operation=Up  start_count=0  cnt_by_val=1  arith_type=Unsigned  n_bits=4  bin_pt=0  load_pin=off  rst=on  en=on  explicit_period=on  period=1  dbl_ovrd=off  use_behavioral_HDL=off  implementation=Fabric  use_rpm=on  block_type=counter
      settings: xl_area=[0, 0, 0, 0, 0, 0, 0]
  payload_count : xbsIndex_r4/Counter  cnt_type=Free Running  cnt_to=Inf  operation=Up  start_count=0  cnt_by_val=1  arith_type=Unsigned  n_bits=8  bin_pt=0  load_pin=off  rst=on  en=on  explicit_period=on  period=1  dbl_ovrd=off  use_behavioral_HDL=off  implementation=Fabric  block_type=counter
      settings: block_version=11.4
  posedge : casper_library_misc/posedge  Tag=Rising Edge Detector  SystemSampleTime=-1
  spead_fsm : xbsIndex_r4/MCode  mfname=spead_fsm  explicit_period=on  period=1  inputsTable={'boundInpExpr'=>['','','','5','','','','',''],'inputs'=>['head_count','num_payload_sent','total_header_len','min_header_len','num_words_sent','payload_len','total_num_payloads','data_valid_in','rst']}  outputsTable={'outputs'=>['head_count_rst','head_count_en','num_payload_rst','num_payload_en','words_sent_rst','words_sent_en','tge_valid','heap_elements','select_data','st'],'suppressOut'=>['off','off','off','off','off','off','off','off','off','off']}  dbl_ovrd=off  enable_stdout=off  enable_debug=off  suppress_output=on  defparams={'min_header_len',5}  hide_port_list={}  block_type=mcode
      settings: block_version=11.4
  words_count : xbsIndex_r4/Counter  cnt_type=Free Running  cnt_to=Inf  operation=Up  start_count=0  cnt_by_val=8  arith_type=Unsigned  n_bits=15  bin_pt=0  load_pin=off  rst=on  en=on  explicit_period=on  period=1  dbl_ovrd=off  use_behavioral_HDL=off  implementation=Fabric  block_type=counter
      settings: block_version=11.4
  data_out : Outport
  data_valid : Outport  Port=2
  eof : Outport  Port=3
  eoh : Outport  Port=4
  wires:
  [eoh] -> payload_cnt1/2
  [reset] -> payload_cnt1/1
  payload_cnt1/1 -> [heap_count]
  payload_cnt5/1 -> Relational/1
  Constant16/1 -> Relational/2
  Relational/1 -> [eoh], eoh/1
  [eof] -> payload_cnt5/2
  [eoh] -> payload_cnt5/1
  [eoh] -> Gateway Out3/1
  [sel_data] -> Mux1/1
  [out_sel] -> Mux1/2
  Mux/1 -> Delay3/1
  Delay3/1 -> [data_out], data_out/1
  Mult/1 -> [heap_offset]
  [pld_len] -> Mult/1
  [num_payload] -> Mult/2
  Delay2/1 -> posedge/1
  Constant15/1 -> spead_fsm/3
  [num_words] -> spead_fsm/4
  [pld_len] -> spead_fsm/5
  Constant8/1 -> spead_fsm/6
  Assert8/1 -> spead_fsm/7
  Assert3/1 -> [reset], spead_fsm/8
  [word_rst] -> Delay2/1
  posedge/1 -> [eof], eof/1
  Gateway Out5/1 -> Scope1/2
  [valid_in] -> Gateway Out5/1
  [num_payload] -> spead_fsm/2
  [out_sel] -> spead_fsm/1
  heap_count/1 -> [out_sel]
  payload_count/1 -> [num_payload]
  words_count/1 -> [num_words]
  Convert/1 -> Concat/6
  [heap_items] -> Convert/1
  spead_fsm/9 -> [sel_data]
  spead_fsm/10 -> [st]
  Mux1/1 -> Mux/1
  Constant20/1 -> Mux1/3
  [data_out] -> Gateway Out4/1
  Gateway Out4/1 -> Scope1/4
  Gateway Out3/1 -> Scope1/6
  Gateway Out1/1 -> Scope1/1
  [data_in] -> Gateway Out1/1
  Reset/1 -> Assert3/1
  [heap_offset] -> Concat1/2
  valid_in/1 -> [valid_in], Assert8/1
  spead_fsm/8 -> [heap_items]
  spead_fsm/7 -> [spead_valid]
  spead_fsm/2 -> [heap_cnt], heap_count/2
  spead_fsm/1 -> heap_count/1
  spead_fsm/4 -> [word_rst], payload_count/2
  spead_fsm/3 -> payload_count/1
  spead_fsm/6 -> words_count/2
  spead_fsm/5 -> words_count/1
  Gateway Out6/1 -> Scope1/5
  Gateway Out2/1 -> Scope1/3
  Concat8/1 -> Mux/9
  Constant14/1 -> Concat8/1
  Assert9/1 -> Concat8/2
  integration size/1 -> Assert9/1
  Concat5/1 -> Mux/7
  Concat6/1 -> Mux/8
  Constant11/1 -> Concat6/1
  Assert7/1 -> Concat6/2
  spectrum counter/1 -> Assert7/1
  Concat9/1 -> Mux/10
  Concat10/1 -> Mux/11
  Concat7/1 -> Mux/12
  Concat1/1 -> Mux/5
  Constant1/1 -> Concat1/1
  [eof] -> Gateway Out6/1
  Delay1/1 -> [valid_out], data_valid/1
  [valid_out] -> Gateway Out2/1
  Packet_length/1 -> Assert4/1
  [spead_valid] -> Delay1/1
  Concat2/1 -> Mux/3
  Assert5/1 -> Concat5/2
  Assert4/1 -> [pld_len], Concat4/2
  Assert2/1 -> [heap_size], Concat3/2
  [heap_count] -> Concat2/2
  heap_size/1 -> Assert2/1
  time_stamp/1 -> Assert5/1
  data_in/1 -> Mux/13, [data_in]
  Constant10/1 -> Concat5/1
  Constant12/1 -> Concat7/1
  Constant13/1 -> Concat2/1
  Constant2/1 -> Concat3/1
  Constant3/1 -> Concat/1
  Constant4/1 -> Concat/2
  Constant5/1 -> Concat/3
  Constant6/1 -> Concat/4
  Constant7/1 -> Concat/5
  Constant9/1 -> Concat4/1
  Concat/1 -> Mux/2
  Concat3/1 -> Mux/4
  Concat4/1 -> Mux/6
  Constant18/1 -> Concat9/1
  mode/1 -> Assert10/1
  Assert10/1 -> Concat9/2
  Constant19/1 -> Concat10/1
  status_bits/1 -> Assert11/1
  Assert11/1 -> Concat10/2
  payload_offset/1 -> Assert12/1
  Assert12/1 -> Concat7/2
